simulink model "sampleModel216"  (R2021b)
settings: Solver=VariableStepAuto  StartTime=0.0  StopTime=10.0  RelTol=1e-3
undefined symbols (not defined in the file or in its folder): DiscIntNeverNeededParam
libraries: simulink x6
settings Model: Creator=user  LastModifiedBy=user

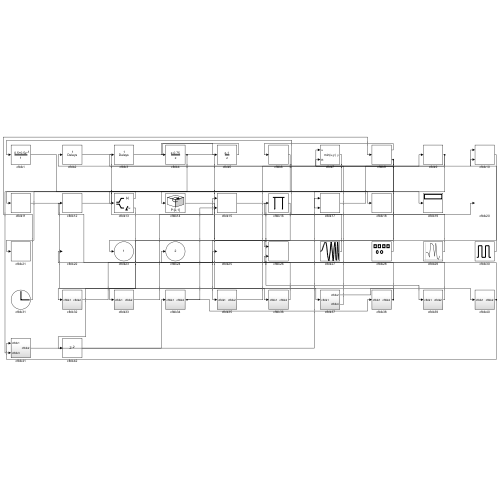
[thumbnail: Simulink's stored preview of the top-level diagram]
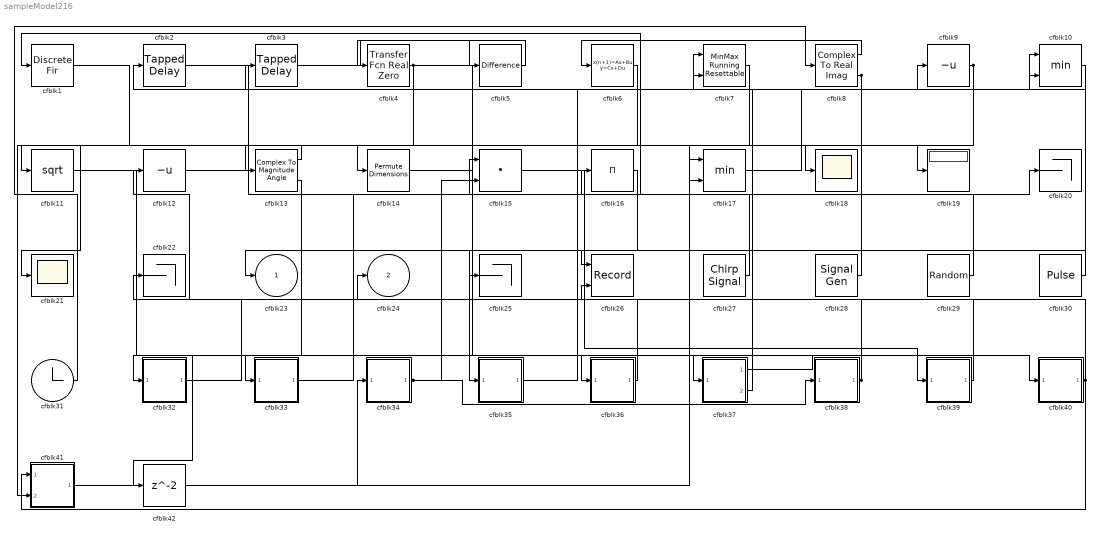
== system sampleModel216 ==
  cfblk1 : DiscreteFir  SampleTime=1
  cfblk10 : MinMax  Inputs=2
  cfblk11 : Sqrt  SaturateOnIntegerOverflow=on
  cfblk12 : UnaryMinus
  cfblk13 : ComplexToMagnitudeAngle
  cfblk14 : PermuteDimensions
  cfblk15 : DotProduct  InputSameDT=on  OutDataTypeStr=Inherit: Inherit via internal rule
  cfblk16 : Product  Inputs=*
  cfblk17 : MinMax  Inputs=2
  cfblk18 : Scope
  cfblk19 : Display
  cfblk2 : simulink/Discrete/Tapped Delay  vinit=0.0  samptime=-1  NumDelays=1  DelayOrder=Oldest  includeCurrent=off
  cfblk20 : Terminator
  cfblk21 : Scope
  cfblk22 : Terminator
  cfblk25 : Terminator
  cfblk26 : Record  FileSettingsInternal="{\"entries\":[{\"content\":{\"excelSettings\":{\"content\":{},\"type\":\"Streamout.ExcelSettings\"}},\"type\":\"Streamout.FileSettingStorage\",\"uuid\":\"aa137edb-8c83-442c-be50-530a3e74da26\"}],\"packageUris\":[\"http://schema.mathworks.com/mf0/streamout_blocks/R2020a\"],\"version\":\"1.0\"}"  Layout=[1 1]  SignalsInternal="{\"entries\":[{\"content\":{\"signals\":[{\"content\":{\"blockPath\":[\"sampleModel216/cfblk26\"],\"channel\":[],\"dimensions\":[1],\"domain\":\"sampleModel216/cfblk26\",\"lineColor\":\"#a2142f\",\"plots\":[1],\"port\":1,\"sid\":[\"\"],\"signalID\":8335,\"signalName\":\"cfblk4\"},\"type\":\"RecordBlkView.Signal\",\"uuid\":\"69c20124-19ff-4eef-a6c2-fd2fba1449b7\"},{\"content\":{\"blockPath\":[\"sampleModel216/cfblk26\"],\"channel\":[],\"dimensions\":[1],\"domain\":\"sampleModel216/cfblk26\",\"lineColor\":\"#139fff\",\"plots\":[1],\"port\":2,\"sid\":[\"\"],\"signalID\":8339,\"signalName\":\"cfblk40\"},\"type\":\"RecordBlkView.Signal\",\"uuid\":\"fc380550-c812-4843-92b8-c1ad71507bdb\"}]},\"type\":\"RecordBlkView.InputSignals\",\"uuid\":\"8e4d784c-5ca3-44ff-a702-21fa2e70ef0c\"}],\"packageUris\":[\"http://schema.mathworks.com/mf0/streamout_blocks/R2020a\"],\"version\":\"1.0\"}"  VisualizationBindings="{\"xyplotplugin\":{\"info\":[{\"series\":[{\"bindingParametersList\":[{\"parameter\":\"X-Axis\",\"signalID\":8335,\"signalName\":\"cfblk4\"},{\"parameter\":\"Y-Axis\",\"signalID\":8339,\"signalName\":\"cfblk40\"}],\"seriesID\":50935}],\"subplotID\":1}]}}"  CompatibilityTag=XY
  cfblk27 : simulink/Sources/Chirp Signal  f1=[981975401.427029]  T=[527231120.705421]  f2=[883080434.445041]
  cfblk28 : SignalGenerator  WaveForm=sawtooth  Amplitude=[-817096306.845178]  Units=rad/sec
  cfblk29 : RandomNumber  Mean=[-17177.912426]  Variance=[55449.262535]  Seed=[361282231.000000]  SampleTime=0.1
  cfblk3 : simulink/Discrete/Tapped Delay  vinit=0.0  samptime=-1  NumDelays=1  DelayOrder=Oldest  includeCurrent=off
  cfblk30 : DiscretePulseGenerator  PulseType=Time based  Amplitude=[627509157.809357]  Period=[95771482.309183]  PulseWidth=5  PhaseDelay=[7.000000]
  cfblk31 : Clock
  cfblk32 : Subsystem
  cfblk33 : Subsystem
  cfblk34 : Subsystem
  cfblk35 : Subsystem
  cfblk36 : Subsystem
  cfblk37 : Subsystem
  cfblk38 : Subsystem
  cfblk39 : Subsystem
  cfblk4 : simulink/Discrete/Transfer Fcn Real Zero  ZeroZ=0.75  ICPrevInput=0.0  DoSatur=off
      settings: SourceProductBaseCode=SL
  cfblk40 : Subsystem
  cfblk41 : Subsystem
  cfblk42 : Delay  SampleTime=1
  cfblk5 : simulink/Discrete/Difference  ICPrevInput=0.0  OutMin=[]  OutMax=[]  OutDataTypeStr=Inherit: Inherit via back propagation  OutDataType=fixdt(1, 16)  OutScaling=2^-10  DoSatur=off
  cfblk6 : DiscreteStateSpace
  cfblk7 : simulink/Math Operations/MinMax Running Resettable  Function=min  vinit=0.0
  cfblk8 : ComplexToRealImag
  cfblk9 : UnaryMinus
  cfblk23 : Outport
  cfblk24 : Outport  Port=2
  wires:
  cfblk11/1 -> cfblk37/1(cfblk1)
  cfblk6/1 -> cfblk14/1
  cfblk41/1(cfblk2) -> cfblk34/1(cfblk1)
  cfblk15/1 -> cfblk39/1(cfblk1)
  cfblk4/1 -> cfblk26/1, cfblk21/1
  cfblk40/1(cfblk2) -> cfblk41/1(cfblk1), cfblk26/2
  cfblk2/1 -> cfblk15/1
  cfblk3/1 -> cfblk5/1
  cfblk27/1 -> cfblk1/1
  cfblk31/1 -> cfblk8/1
  cfblk16/1 -> cfblk23/1
  cfblk33/1(cfblk2) -> cfblk20/1
  cfblk39/1(cfblk2) -> cfblk24/1
  cfblk38/1(cfblk2) -> cfblk32/1(cfblk1), cfblk12/1
  cfblk12/1 -> cfblk18/1
  cfblk8/1 -> cfblk6/1
  cfblk36/1(cfblk2) -> cfblk22/1
  cfblk8/2 -> cfblk35/1(cfblk1), cfblk3/1, cfblk17/2
  cfblk10/1 -> cfblk33/1(cfblk1)
  cfblk14/1 -> cfblk36/1(cfblk1)
  cfblk34/1(cfblk2) -> cfblk38/1(cfblk1), cfblk15/2
  cfblk35/1(cfblk2) -> cfblk10/1
  cfblk32/1(cfblk2) -> cfblk25/1
  cfblk30/1 -> cfblk10/2
  cfblk37/1(cfblk2) -> cfblk40/1(cfblk1)
  cfblk7/1 -> cfblk41/2(cfblk3)
  cfblk37/2(cfblk4) -> cfblk7/1
  cfblk17/1 -> cfblk9/1
  cfblk13/1 -> cfblk11/1
  cfblk29/1 -> cfblk16/1
  cfblk5/1 -> cfblk4/1
  cfblk28/1 -> cfblk2/1
  cfblk1/1 -> cfblk19/1
  cfblk9/1 -> cfblk7/2, cfblk13/1
  cfblk13/2 -> cfblk42/1
  cfblk42/1 -> cfblk17/1

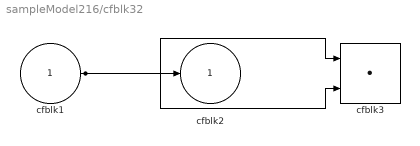
== system sampleModel216/cfblk32 ==
  cfblk1 : Inport
  cfblk3 : DotProduct  InputSameDT=on  OutDataTypeStr=Inherit: Inherit via internal rule
  cfblk2 : Outport
  wires:
  cfblk1/1 -> cfblk2/1, cfblk3/1, cfblk3/2

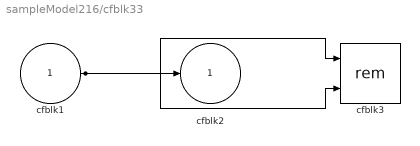
== system sampleModel216/cfblk33 ==
  cfblk1 : Inport
  cfblk3 : Math  Operator=rem  SaturateOnIntegerOverflow=on
  cfblk2 : Outport
  wires:
  cfblk1/1 -> cfblk2/1, cfblk3/1, cfblk3/2

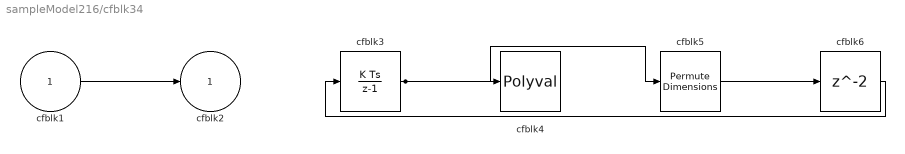
== system sampleModel216/cfblk34 ==
  cfblk1 : Inport
  cfblk3 : DiscreteIntegrator  ICPrevOutput=DiscIntNeverNeededParam  ICPrevScaledInput=DiscIntNeverNeededParam
  cfblk4 : Polyval  Coefs=[ +2.081618890e-019, -1.441693666e-014, +4.719686976e-010, -8.536869453e-006, +1.621573104e-001, -8.087801117e+001 ]
  cfblk5 : PermuteDimensions
  cfblk6 : Delay  SampleTime=1
  cfblk2 : Outport
  wires:
  cfblk3/1 -> cfblk5/1, cfblk4/1
  cfblk1/1 -> cfblk2/1
  cfblk5/1 -> cfblk6/1
  cfblk6/1 -> cfblk3/1

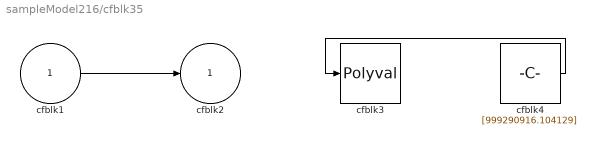
== system sampleModel216/cfblk35 ==
  cfblk1 : Inport
  cfblk3 : Polyval  Coefs=[ +2.081618890e-019, -1.441693666e-014, +4.719686976e-010, -8.536869453e-006, +1.621573104e-001, -8.087801117e+001 ]
  cfblk4 : Constant  Value=[999290916.104129]  SampleTime=1
  cfblk2 : Outport
  wires:
  cfblk1/1 -> cfblk2/1
  cfblk4/1 -> cfblk3/1

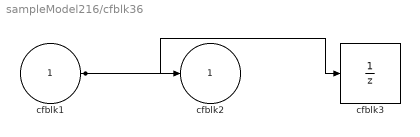
== system sampleModel216/cfblk36 ==
  cfblk1 : Inport
  cfblk3 : UnitDelay  HasFrameUpgradeWarning=on
  cfblk2 : Outport
  wires:
  cfblk1/1 -> cfblk2/1, cfblk3/1

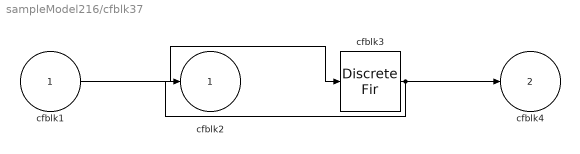
== system sampleModel216/cfblk37 ==
  cfblk1 : Inport
  cfblk3 : DiscreteFir  SampleTime=1
  cfblk2 : Outport
  cfblk4 : Outport  Port=2
  wires:
  cfblk1/1 -> cfblk3/1
  cfblk3/1 -> cfblk2/1, cfblk4/1

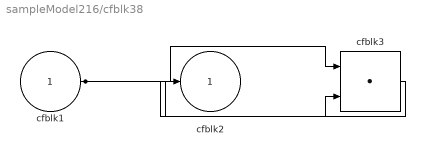
== system sampleModel216/cfblk38 ==
  cfblk1 : Inport
  cfblk3 : DotProduct  InputSameDT=on  OutDataTypeStr=Inherit: Inherit via internal rule
  cfblk2 : Outport
  wires:
  cfblk1/1 -> cfblk3/1, cfblk3/2
  cfblk3/1 -> cfblk2/1

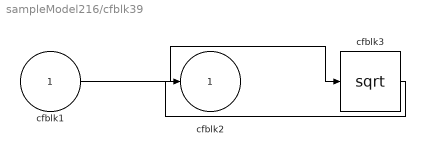
== system sampleModel216/cfblk39 ==
  cfblk1 : Inport
  cfblk3 : Sqrt  SaturateOnIntegerOverflow=on
  cfblk2 : Outport
  wires:
  cfblk1/1 -> cfblk3/1
  cfblk3/1 -> cfblk2/1

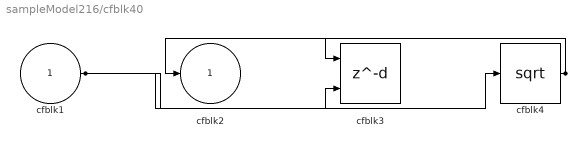
== system sampleModel216/cfblk40 ==
  cfblk1 : Inport
  cfblk3 : Delay  DelayLengthSource=Input port  SampleTime=1
      settings: InputPortMap=u0,p1
  cfblk4 : Sqrt  SaturateOnIntegerOverflow=on
  cfblk2 : Outport
  wires:
  cfblk4/1 -> cfblk2/1, cfblk3/1
  cfblk1/1 -> cfblk4/1, cfblk3/2

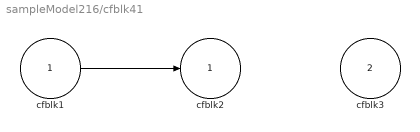
== system sampleModel216/cfblk41 ==
  cfblk1 : Inport
  cfblk3 : Inport  Port=2
  cfblk2 : Outport
  wires:
  cfblk1/1 -> cfblk2/1
